simulink model "doc_phasetree"  (Simulink 4.00)
settings: Solver=ode45  StartTime=0.0  StopTime=10.0  RelTol=1e-3
undefined symbols (not defined in the file): s, slcm
libraries: commdigbbndcpm2 x1, dspsrcs3 x1
settings Model: RequirementInfo=9  Creator=tdelve  LastModifiedBy=agaltman  BlockReductionOpt=off

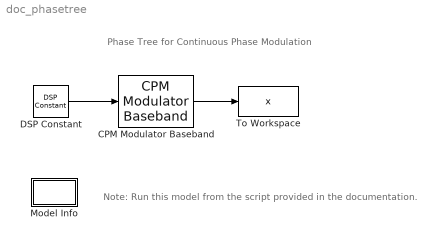
== system doc_phasetree ==
  note: Phase Tree for Continuous Phase Modulation
  note: Note: Run this model from the script provided in the documentation.
  CPM Modulator Baseband : commdigbbndcpm2/CPM Modulator Baseband  Mnum=2  inputType=Integer  mappingType=Binary  modIdx=2/3  pulseShape=Raised Cosine  BT=0.3  rollOff=0.2  pulseLength=2  preHistory=1  phaseOffset=0  samplesPerSymbol=8
  DSP Constant : dspsrcs3/DSP Constant  Value=s  InterpretAs1D=off  SampleMode=Discrete  Ts=1  FramebasedOutput=on
  Model Info : Subsystem  LoadFcn=slcm LoadBlock;  InitFcn=slcm('UpdateAllCMBlocksInThisModelInit')  mask(CMBlock){InitialSaveTempField=, InitialBlockCM=none, BlockCM=none, Frame=on, SaveTempField=, DisplayStringWithTags=Info, MaskDisplayString=Info, HorizontalTextAlignment=Center, LeftAlignmentValue=0.5, SourceBlockDiagram=doc_phasetree, TagMaxNumber=20, CMTag1=, CMTag2=, CMTag3=, CMTag4=, CMTag5=, CMTag6=, CMTag7=, CMTag8=, CMTag9=, CMTag10=, CMTag11=, CMTag12=, CMTag13=, CMTag14=, CMTag15=, CMTag16=, CMTag17=, CMTag18=, CMTag19=, CMTag20=}
      mask help: This block allows revision control information to be displayed within the model.
      settings: CopyFcn=slcm CopyBlock;  DeleteFcn=slcm Cancel;  PostSaveFcn=slcm('UpdateAllCMBlocksInThisModel')  NameChangeFcn=slcm Rename;  OpenFcn=commdemohelp;  RTWFcnNameOpts=Auto  RTWFileNameOpts=Auto
      mask Display: text(str2num(LeftAlignmentValue), 0.5, MaskDisplayString, 'HorizontalAlignment', HorizontalTextAlignment)
  To Workspace : ToWorkspace  VariableName=x  SampleTime=-1  SaveFormat=Array
  wires:
  CPM Modulator Baseband/1 -> To Workspace/1
  DSP Constant/1 -> CPM Modulator Baseband/1

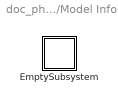
== system doc_phasetree/Model Info ==
  EmptySubsystem : Subsystem
      settings: RTWFcnNameOpts=Auto  RTWFileNameOpts=Auto

== system doc_phasetree/Model Info/EmptySubsystem ==
